simulink model "Simulink_Simulation"  (R2021a)
settings: Solver=VariableStepAuto  StartTime=0.0  StopTime=10.0  RelTol=1e-3
settings Model: Creator=nicol  LastModifiedBy=nicol

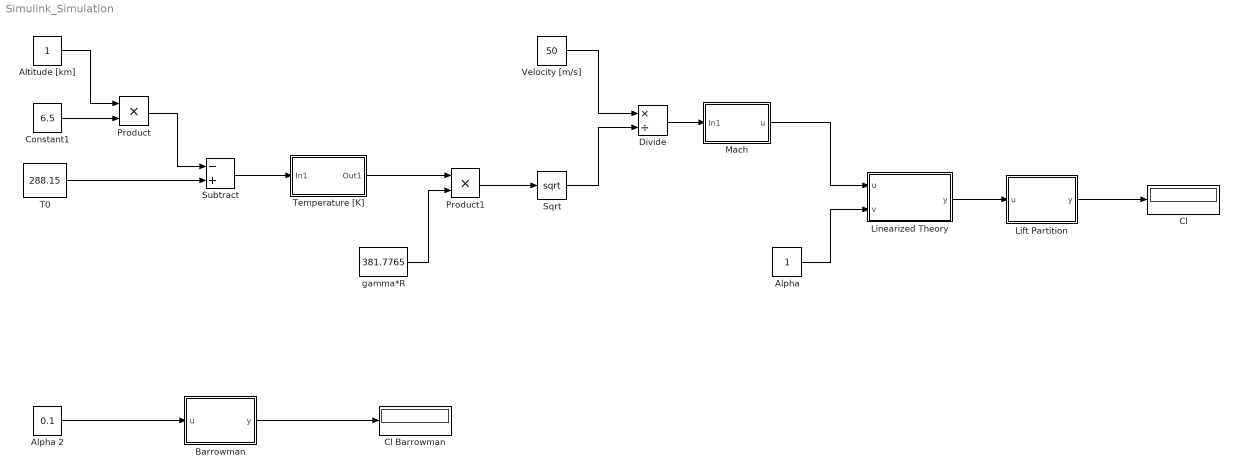
== system Simulink_Simulation ==
  Alpha : Constant
  Alpha 2 : Constant  Value=0.1
  Altitude [km] : Constant
  Barrowman : MATLAB Function  TreatAsAtomicUnit=on
  Cl : Display
  Cl Barrowman : Display
  Constant1 : Constant  Value=6.5
  Divide : Product  Inputs=*/
  Lift Partition : MATLAB Function  TreatAsAtomicUnit=on
  Linearized Theory : MATLAB Function  TreatAsAtomicUnit=on
  Mach : Subsystem
  Product : Product
  Product1 : Product
  Sqrt : Sqrt  SaturateOnIntegerOverflow=on
  Subtract : Sum  Inputs=-+
  T0 : Constant  Value=288.15
  Temperature [K] : Subsystem
  Velocity [m/s] : Constant  Value=50
  gamma*R : Constant  Value=381.7765
  wires:
  Linearized Theory/1(y) -> Lift Partition/1(u)
  Alpha/1 -> Linearized Theory/2(v)
  Lift Partition/1(y) -> Cl/1
  T0/1 -> Subtract/2
  Product/1 -> Subtract/1
  Altitude [km]/1 -> Product/1
  Constant1/1 -> Product/2
  Subtract/1 -> Temperature [K]/1(In1)
  Velocity [m/s]/1 -> Divide/1
  Sqrt/1 -> Divide/2
  Temperature [K]/1(Out1) -> Product1/1
  Product1/1 -> Sqrt/1
  gamma*R/1 -> Product1/2
  Divide/1 -> Mach/1(In1)
  Mach/1(u) -> Linearized Theory/1(u)
  Alpha 2/1 -> Barrowman/1(u)
  Barrowman/1(y) -> Cl Barrowman/1

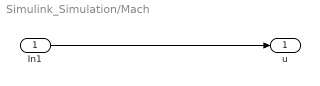
== system Simulink_Simulation/Mach ==
  In1 : Inport
  u : Outport
  wires:
  In1/1 -> u/1

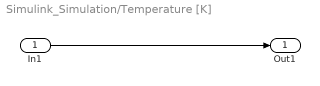
== system Simulink_Simulation/Temperature [K] ==
  In1 : Inport
  Out1 : Outport
  wires:
  In1/1 -> Out1/1

== matlab function Simulink_Simulation/Linearized Theory ==
  data: u input; y output; v input
function y = fcn(u,v)
% First method, linearized theory for a thin plate
y = ((2*pi*(v*2*pi)/360)/(sqrt(1-u^2)))*13500/(2*pi*52^2);

== matlab function Simulink_Simulation/Barrowman ==
  data: u input; y output
function y = fcn(u)
% Barrowman
C_N_nose = 2;
r = 52;
LF = 119;
CR = 200;
CT = 70;
s = 100;
n = 4;
interference_factor = 1+(r/(s+r));
C_N_fins = (4*n*(s/(2*r))^2)/(1+sqrt(1+((2*LF)/(CR+CT))^2));
C_N_fins_interf = C_N_fins * interference_factor;
y = (C_N_nose+C_N_fins_interf)*cos(u*2*pi/360).*((u*2*pi)/360);

== matlab function Simulink_Simulation/Lift Partition ==
  data: u input; y output
function y = fcn(u)
% Second method, lift partition
y = u*2;
